simulink model "SimulinkRLC"  (R2023b)
settings: Solver=VariableStepAuto  StartTime=0.0  StopTime=0.003  RelTol=1e-3
settings Model: LastModifiedBy=ZBOOK 15 G7

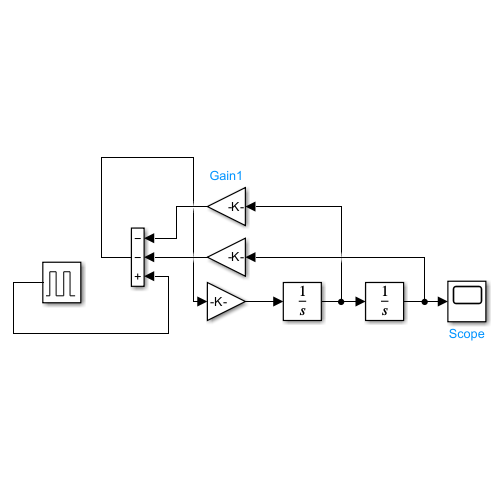
[thumbnail: Simulink's stored preview of the top-level diagram]
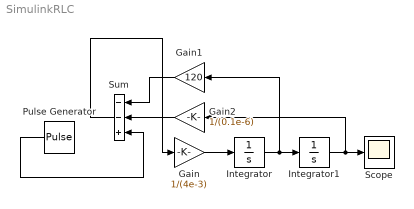
== system SimulinkRLC ==
  Gain : Gain  Gain=1/(4e-3)
  Gain1 : Gain  Gain=120
  Gain2 : Gain  Gain=1/(0.1e-6)
  Integrator : Integrator
  Integrator1 : Integrator
  Pulse Generator : DiscretePulseGenerator  PulseType=Time based  Amplitude=12  Period=0.002  PulseWidth=50
  Scope : Scope
  Sum : Sum  Inputs=--+
  wires:
  Integrator/1 -> Gain1/1, Integrator1/1
  Gain/1 -> Integrator/1
  Integrator1/1 -> Gain2/1, Scope/1
  Gain2/1 -> Sum/2
  Pulse Generator/1 -> Sum/3
  Gain1/1 -> Sum/1
  Sum/1 -> Gain/1
